simulink model "sampleModel283"  (R2021b)
settings: Solver=VariableStepAuto  StartTime=0.0  StopTime=10.0  RelTol=1e-3
undefined symbols (not defined in the file or in its folder): DiscIntNeverNeededParam
libraries: simulink x9, slpidlib x3
settings Model: Creator=user  LastModifiedBy=user

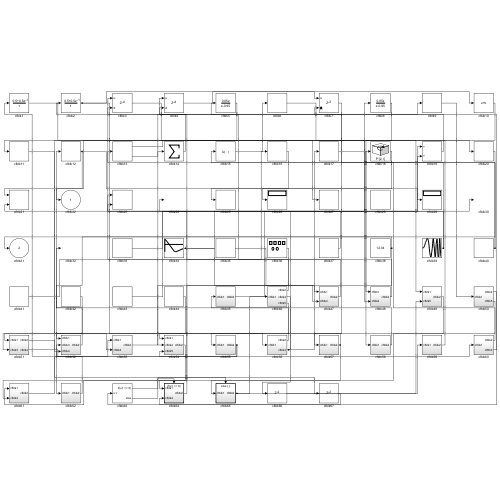
[thumbnail: Simulink's stored preview of the top-level diagram]
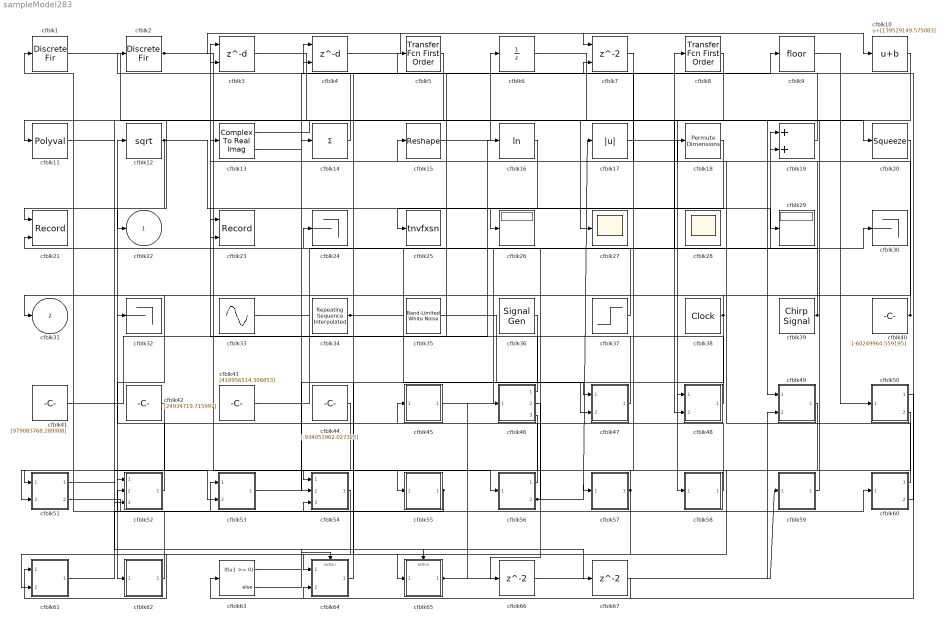
== system sampleModel283 ==
  cfblk1 : DiscreteFir  SampleTime=1
  cfblk10 : Bias  Bias=[139529149.575083]
  cfblk11 : Polyval  Coefs=[ +2.081618890e-019, -1.441693666e-014, +4.719686976e-010, -8.536869453e-006, +1.621573104e-001, -8.087801117e+001 ]
  cfblk12 : Sqrt  SaturateOnIntegerOverflow=on
  cfblk13 : ComplexToRealImag
  cfblk14 : Sum  Inputs=+
  cfblk15 : Reshape
  cfblk16 : Math  Operator=log  SaturateOnIntegerOverflow=on
  cfblk17 : Abs
  cfblk18 : PermuteDimensions
  cfblk19 : Sum
  cfblk2 : DiscreteFir  SampleTime=1
  cfblk20 : Squeeze
  cfblk21 : Record  FileSettingsInternal="{\"entries\":[{\"content\":{\"excelSettings\":{\"content\":{},\"type\":\"Streamout.ExcelSettings\"}},\"type\":\"Streamout.FileSettingStorage\",\"uuid\":\"8694a5bb-1d16-4ad7-950e-c35a4b4d7b5d\"}],\"packageUris\":[\"http://schema.mathworks.com/mf0/streamout_blocks/R2020a\"],\"version\":\"1.0\"}"  Layout=[1 1]  SignalsInternal="{\"entries\":[{\"content\":{\"signals\":[{\"content\":{\"blockPath\":[\"sampleModel283/cfblk21\"],\"channel\":[],\"dimensions\":[1],\"domain\":\"sampleModel283/cfblk21\",\"lineColor\":\"#a2142f\",\"plots\":[1],\"port\":1,\"sid\":[\"\"],\"signalID\":12100,\"signalName\":\"cfblk12\"},\"type\":\"RecordBlkView.Signal\",\"uuid\":\"68d03bc7-fcef-4d0a-a321-f31d8b845c33\"},{\"content\":{\"blockPath\":[\"sampleModel283/cfblk21\"],\"channel\":[],\"dimensions\":[1],\"domain\":\"sampleModel283/cfblk21\",\"lineColor\":\"#139fff\",\"plots\":[1],\"port\":2,\"sid\":[\"\"],\"signalID\":12104,\"signalName\":\"cfblk37\"},\"type\":\"RecordBlkView.Signal\",\"uuid\":\"b222a0ad-5142-49e8-822e-f4ea90e28b72\"}]},\"type\":\"RecordBlkView.InputSignals\",\"uuid\":\"76179848-0323-487f-86f4-e1829027746c\"}],\"packageUris\":[\"http://schema.mathworks.com/mf0/streamout_blocks/R2020a\"],\"version\":\"1.0\"}"  VisualizationBindings="{\"xyplotplugin\":{\"info\":[{\"series\":[{\"bindingParametersList\":[{\"parameter\":\"X-Axis\",\"signalID\":12100,\"signalName\":\"cfblk12\"},{\"parameter\":\"Y-Axis\",\"signalID\":12104,\"signalName\":\"cfblk37\"}],\"seriesID\":11155}],\"subplotID\":1}]}}"  CompatibilityTag=XY
  cfblk23 : Record  FileSettingsInternal="{\"entries\":[{\"content\":{\"excelSettings\":{\"content\":{},\"type\":\"Streamout.ExcelSettings\"}},\"type\":\"Streamout.FileSettingStorage\",\"uuid\":\"90ddd849-edd4-4e39-a333-4208290193cd\"}],\"packageUris\":[\"http://schema.mathworks.com/mf0/streamout_blocks/R2020a\"],\"version\":\"1.0\"}"  Layout=[1 1]  SignalsInternal="{\"entries\":[{\"content\":{\"signals\":[{\"content\":{\"blockPath\":[\"sampleModel283/cfblk23\"],\"channel\":[],\"dimensions\":[1],\"domain\":\"sampleModel283/cfblk23\",\"lineColor\":\"#a2142f\",\"plots\":[1],\"port\":1,\"sid\":[\"\"],\"signalID\":12108,\"signalName\":\"cfblk39\"},\"type\":\"RecordBlkView.Signal\",\"uuid\":\"9c057a92-301d-4b39-ab38-061aa18ef5d9\"},{\"content\":{\"blockPath\":[\"sampleModel283/cfblk23\"],\"channel\":[],\"dimensions\":[1],\"domain\":\"sampleModel283/cfblk23\",\"lineColor\":\"#139fff\",\"plots\":[1],\"port\":2,\"sid\":[\"\"],\"signalID\":12112,\"signalName\":\"cfblk56:2\"},\"type\":\"RecordBlkView.Signal\",\"uuid\":\"a825d14d-2c29-4b3e-948f-2c2b4e7bd86f\"}]},\"type\":\"RecordBlkView.InputSignals\",\"uuid\":\"38af6987-c0c5-4704-b1ef-83ad3136d3ff\"}],\"packageUris\":[\"http://schema.mathworks.com/mf0/streamout_blocks/R2020a\"],\"version\":\"1.0\"}"  VisualizationBindings="{\"xyplotplugin\":{\"info\":[{\"series\":[{\"bindingParametersList\":[{\"parameter\":\"X-Axis\",\"signalID\":12108,\"signalName\":\"cfblk39\"},{\"parameter\":\"Y-Axis\",\"signalID\":12112,\"signalName\":\"cfblk56:2\"}],\"seriesID\":64880}],\"subplotID\":1}]}}"  CompatibilityTag=XY
  cfblk24 : Terminator
  cfblk25 : ToWorkspace  VariableName=tnvfxsn  SaveFormat=Timeseries  SampleTime=-1
  cfblk26 : Display
  cfblk27 : Scope
  cfblk28 : Scope
      settings: Floating=on
  cfblk29 : Display
  cfblk3 : Delay  DelayLengthSource=Input port  SampleTime=1
      settings: InputPortMap=u0,p1
  cfblk30 : Terminator
  cfblk32 : Terminator
  cfblk33 : Sin  Amplitude=[128819876.540734]  Bias=[698200433.289732]  SampleTime=0
  cfblk34 : simulink/Sources/Repeating Sequence Interpolated  OutValues=[457661850.297885, 290690144.508280, -581221308.548181, -642320160.638465, -356637687.568462]  TimeValues=[0 0.1 0.5 0.6 1].'  LookUpMeth=Use Input Below  tsamp=0.01  OutMin=[]  OutMax=[]  OutDataTypeStr=double  OutputDataTypeScalingMode=double  OutDataType=fixdt(0,8)  OutScaling=2^-10
  cfblk35 : simulink/Sources/Band-Limited White Noise  Cov=[1006841987.893803]  Ts=0.1  seed=[5581259503.000000]
  cfblk36 : SignalGenerator  WaveForm=square  Amplitude=[368174655.835128]  Units=rad/sec
  cfblk37 : Step  Time=[38.000000]  Before=[-937039488.309373]  After=[-569842712.243944]  SampleTime=0
  cfblk38 : DigitalClock
  cfblk39 : simulink/Sources/Chirp Signal  f1=[685027736.106860]  T=[-403921099.241479]  f2=[736095362.275255]
  cfblk4 : Delay  DelayLengthSource=Input port  SampleTime=1
      settings: InputPortMap=u0,p1
  cfblk40 : Constant  Value=[-60249964.559195]  SampleTime=1
  cfblk41 : Constant  Value=[979083768.289908]  SampleTime=1
  cfblk42 : Constant  Value=[24934719.715997]  SampleTime=1
  cfblk43 : Constant  Value=[418956514.306853]  SampleTime=1
  cfblk44 : Constant  Value=[-934051962.027325]  SampleTime=1
  cfblk45 : Subsystem
  cfblk46 : Subsystem
  cfblk47 : Subsystem
  cfblk48 : Subsystem
  cfblk49 : Subsystem
  cfblk5 : simulink/Discrete/Transfer Fcn First Order  PoleZ=0.95  ICPrevOutput=0.0  DoSatur=off
  cfblk50 : Subsystem
  cfblk51 : Subsystem
  cfblk52 : Subsystem
  cfblk53 : Subsystem
  cfblk54 : Subsystem
  cfblk55 : Subsystem
  cfblk56 : Subsystem
  cfblk57 : Subsystem
  cfblk58 : Subsystem
  cfblk59 : Subsystem
  cfblk6 : UnitDelay  HasFrameUpgradeWarning=on
  cfblk60 : Subsystem
  cfblk61 : Subsystem
  cfblk62 : Subsystem
  cfblk63 : If  IfExpression=u1 >= 0  SampleTime=1
  cfblk64 : Subsystem  TreatAsAtomicUnit=on
  cfblk65 : Subsystem  TreatAsAtomicUnit=on
  cfblk66 : Delay  SampleTime=1
  cfblk67 : Delay  SampleTime=1
  cfblk7 : Delay  ShowEnablePort=on  SampleTime=1
      settings: InputPortMap=u0,e6
  cfblk8 : simulink/Discrete/Transfer Fcn First Order  PoleZ=0.95  ICPrevOutput=0.0  DoSatur=off
  cfblk9 : Rounding
  cfblk22 : Outport
  cfblk31 : Outport  Port=2
  wires:
  cfblk18/1 -> cfblk25/1
  cfblk17/1 -> cfblk58/1(cfblk1)
  cfblk44/1 -> cfblk54/1(cfblk1)
  cfblk49/1(cfblk2) -> cfblk65/1(cfblk1)
  cfblk12/1 -> cfblk21/1, cfblk29/1
  cfblk59/1(cfblk2) -> cfblk11/1
  cfblk2/1 -> cfblk56/1(cfblk1), cfblk7/1
  cfblk9/1 -> cfblk50/1(cfblk1)
  cfblk45/1(cfblk2) -> cfblk30/1
  cfblk50/1(cfblk2) -> cfblk63/1
  cfblk4/1 -> cfblk10/1
  cfblk56/1(cfblk2) -> cfblk45/1(cfblk1)
  cfblk53/1(cfblk2) -> cfblk14/1
  cfblk42/1 -> cfblk62/1(cfblk1)
  cfblk52/1(cfblk2) -> cfblk12/1
  cfblk58/1(cfblk2) -> cfblk32/1
  cfblk47/1(cfblk2) -> cfblk3/1
  cfblk56/2(cfblk4) -> cfblk17/1, cfblk23/2
  cfblk54/1(cfblk2) -> cfblk61/1(cfblk1)
  cfblk46/1(cfblk2) -> cfblk4/1
  cfblk33/1 -> cfblk19/1
  cfblk8/1 -> cfblk48/1(cfblk1)
  cfblk7/1 -> cfblk57/1(cfblk1)
  cfblk34/1 -> cfblk19/2, cfblk47/2(cfblk4)
  cfblk36/1 -> cfblk64/1(cfblk1)
  cfblk60/1(cfblk2) -> cfblk18/1
  cfblk40/1 -> cfblk13/1, cfblk7/2
  cfblk64/1(cfblk2) -> cfblk24/1
  cfblk15/1 -> cfblk6/1
  cfblk16/1 -> cfblk26/1
  cfblk65/1(cfblk2) -> cfblk59/1(cfblk1), cfblk46/1(cfblk1)
  cfblk61/1(cfblk2) -> cfblk60/1(cfblk1)
  cfblk6/1 -> cfblk49/1(cfblk1)
  cfblk57/1(cfblk2) -> cfblk51/1(cfblk1), cfblk61/2(cfblk4)
  cfblk37/1 -> cfblk21/2
  cfblk1/1 -> cfblk48/2(cfblk4)
  cfblk38/1 -> cfblk31/1, cfblk54/2(cfblk4)
  cfblk20/1 -> cfblk52/1(cfblk1)
  cfblk3/1 -> cfblk27/1
  cfblk51/2(cfblk4) -> cfblk53/1(cfblk1)
  cfblk5/1 -> cfblk22/1
  cfblk55/1(cfblk2) -> cfblk52/2(cfblk3), cfblk54/3(cfblk5)
  cfblk48/1(cfblk2) -> cfblk15/1
  cfblk11/1 -> cfblk53/2(cfblk4)
  cfblk14/1 -> cfblk4/2
  cfblk60/2(cfblk3) -> cfblk3/2
  cfblk62/1(cfblk2) -> cfblk1/1
  cfblk19/1 -> cfblk2/1
  cfblk43/1 -> cfblk8/1
  cfblk46/3(cfblk5) -> cfblk51/2(cfblk3)
  cfblk41/1 -> cfblk16/1
  cfblk50/2(cfblk5) -> cfblk55/1(cfblk1)
  cfblk10/1 -> cfblk52/3(cfblk4)
  cfblk13/1 -> cfblk20/1
  cfblk39/1 -> cfblk23/1, cfblk5/1
  cfblk35/1 -> cfblk47/1(cfblk1)
  cfblk13/2 -> cfblk9/1
  cfblk63/1 -> cfblk64/Action
  cfblk63/2 -> cfblk65/Action
  cfblk46/2(cfblk4) -> cfblk66/1
  cfblk66/1 -> cfblk49/2(cfblk5)
  cfblk51/1(cfblk2) -> cfblk67/1
  cfblk67/1 -> cfblk64/2(cfblk4)

== system sampleModel283/cfblk45 ==
  cfblk1 : Inport
  cfblk3 : DiscreteFir  SampleTime=1
  cfblk2 : Outport
  wires:
  cfblk1/1 -> cfblk3/1
  cfblk3/1 -> cfblk2/1

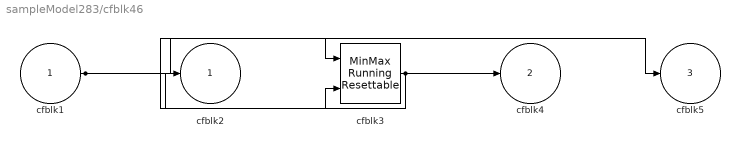
== system sampleModel283/cfblk46 ==
  cfblk1 : Inport
  cfblk3 : simulink/Math Operations/MinMax Running Resettable  Function=min  vinit=0.0
  cfblk2 : Outport
  cfblk4 : Outport  Port=2
  cfblk5 : Outport  Port=3
  wires:
  cfblk1/1 -> cfblk3/1, cfblk3/2, cfblk5/1
  cfblk3/1 -> cfblk2/1, cfblk4/1

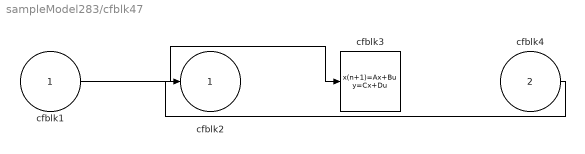
== system sampleModel283/cfblk47 ==
  cfblk1 : Inport
  cfblk4 : Inport  Port=2
  cfblk3 : DiscreteStateSpace
  cfblk2 : Outport
  wires:
  cfblk1/1 -> cfblk3/1
  cfblk4/1 -> cfblk2/1

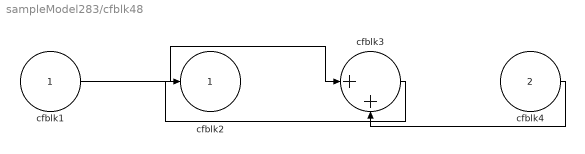
== system sampleModel283/cfblk48 ==
  cfblk1 : Inport
  cfblk4 : Inport  Port=2
  cfblk3 : Sum  Inputs=|++
  cfblk2 : Outport
  wires:
  cfblk1/1 -> cfblk3/1
  cfblk3/1 -> cfblk2/1
  cfblk4/1 -> cfblk3/2

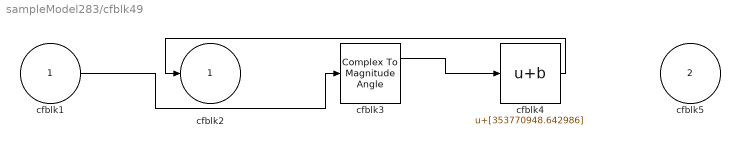
== system sampleModel283/cfblk49 ==
  cfblk1 : Inport
  cfblk5 : Inport  Port=2
  cfblk3 : ComplexToMagnitudeAngle
  cfblk4 : Bias  Bias=[353770948.642986]
  cfblk2 : Outport
  wires:
  cfblk4/1 -> cfblk2/1
  cfblk1/1 -> cfblk3/1
  cfblk3/1 -> cfblk4/1

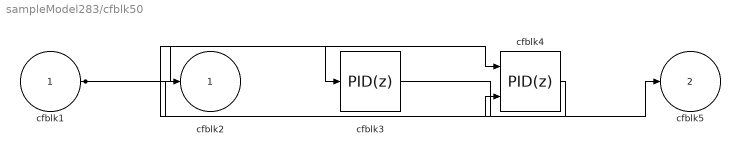
== system sampleModel283/cfblk50 ==
  cfblk1 : Inport
  cfblk3 : slpidlib/PID Controller  Controller=PID  Form=Parallel  TimeDomain=Discrete-time  UseExternalTs=off  SampleTime=1  IntegratorMethod=Forward Euler  FilterMethod=Forward Euler  ControllerParametersSource=internal  P=1  I=1  D=0  UseFilter=on  N=100  TunerSelectOption=Transfer Function Based (PID Tuner App)  InitialConditionSource=internal  InitialConditionForIntegrator=0  InitialConditionForFilter=0  DifferentiatorICPrevScaledInput=0  ExternalReset=none  TrackingMode=off  Kt=1  LimitOutput=off  SatLimitsSource=internal  UpperSaturationLimit=inf  LowerSaturationLimit=-inf  LinearizeAsGain=off  AntiWindupMode=none  Kb=1  POutMin=[]  POutMax=[]  IOutMin=[]  IOutMax=[]  DOutMin=[]  DOutMax=[]  NOutMin=[]  NOutMax=[]  SumOutMin=[]  SumOutMax=[]  SaturationOutMin=[]  SaturationOutMax=[]  PParamMin=[]  PParamMax=[]  IParamMin=[]  IParamMax=[]  DParamMin=[]  DParamMax=[]  NParamMin=[]  NParamMax=[]  KbParamMin=[]  KbParamMax=[]  KtParamMin=[]  KtParamMax=[]  KbOutMin=[]  KbOutMax=[]  KtOutMin=[]  KtOutMax=[]  IntegratorOutMin=[]  IntegratorOutMax=[]  FilterOutMin=[]  FilterOutMax=[]  SumI1OutMin=[]  SumI1OutMax=[]  SumI2OutMin=[]  SumI2OutMax=[]  SumI3OutMin=[]  SumI3OutMax=[]  SumI4OutMin=[]  SumI4OutMax=[]  SumDOutMin=[]  SumDOutMax=[]  DifferentiatorOutMin=[]  DifferentiatorOutMax=[]  FilterDiffOutCoefMin=[]  FilterDiffOutCoefMax=[]  ReciprocalOutMin=[]  ReciprocalOutMax=[]  SumDenOutMin=[]  SumDenOutMax=[]  SumNumOutMin=[]  SumNumOutMax=[]  DivideOutMin=[]  DivideOutMax=[]  UdiffTsProdOutMin=[]  UdiffTsProdOutMax=[]  NTsProdOutMin=[]  NTsProdOutMax=[]  UintegralTsProdOutMin=[]  UintegralTsProdOutMax=[]  UngainTsProdOutMin=[]  UngainTsProdOutMax=[]  IntegratorContinuousStateAttributes=''  IntegratorStateMustResolveToSignalObject=off  IntegratorRTWStateStorageClass=Auto  FilterContinuousStateAttributes=''  FilterStateMustResolveToSignalObject=off  FilterRTWStateStorageClass=Auto  ParallelPVariant=InternalParameters  IdealPVariant=Disabled  IVariant=InternalParameters  DVariant=InternalParameters  IntegratorVariant=Discrete  SatVariant=Disabled  AWVariant=Passthrough  PCopyVariant=Disabled  TRVariant=Disabled  FdbkBlocksVariant=Forward  IdealPFdbkVariant=Disabled  SatFdbkVariant=Disabled  DerivativeFilterVariant=ForwardEulerFilter  NVariant=InternalParameters  NCopyVariant=Disabled  FilterICVariant=InternalICsFilter  IntegratorICVariant=InternalICs  ExternalResetVariant=Disabled  TRSumVariant=Passthrough  SumFdbkVariant=Disabled  SumVariant=Sum_PID  TsampFilterVariant=InternalTs  TsampNgainVariant=Passthrough  TsampIntegralVariant=Passthrough  ExternalSaturationOutDataTypeStr=Inherit: Same as second input
  cfblk4 : slpidlib/PID Controller (2DOF)  Controller=PID  Form=Parallel  TimeDomain=Discrete-time  UseExternalTs=off  SampleTime=1  IntegratorMethod=Forward Euler  FilterMethod=Forward Euler  ControllerParametersSource=internal  P=1  I=1  D=0  UseFilter=on  N=100  b=1  c=1  TunerSelectOption=Transfer Function Based (PID Tuner App)  InitialConditionSource=internal  InitialConditionForIntegrator=0  InitialConditionForFilter=0  DifferentiatorICPrevScaledInput=0  ExternalReset=none  TrackingMode=off  Kt=1  LimitOutput=off  SatLimitsSource=internal  UpperSaturationLimit=inf  LowerSaturationLimit=-inf  LinearizeAsGain=off  AntiWindupMode=none  Kb=1  POutMin=[]  POutMax=[]  IOutMin=[]  IOutMax=[]  DOutMin=[]  DOutMax=[]  NOutMin=[]  NOutMax=[]  bOutMin=[]  bOutMax=[]  cOutMin=[]  cOutMax=[]  SumOutMin=[]  SumOutMax=[]  SaturationOutMin=[]  SaturationOutMax=[]  PParamMin=[]  PParamMax=[]  IParamMin=[]  IParamMax=[]  DParamMin=[]  DParamMax=[]  NParamMin=[]  NParamMax=[]  bParamMin=[]  bParamMax=[]  cParamMin=[]  cParamMax=[]  KbParamMin=[]  KbParamMax=[]  KtParamMin=[]  KtParamMax=[]  KbOutMin=[]  KbOutMax=[]  KtOutMin=[]  KtOutMax=[]  IntegratorOutMin=[]  IntegratorOutMax=[]  FilterOutMin=[]  FilterOutMax=[]  SumI1OutMin=[]  SumI1OutMax=[]  SumI2OutMin=[]  SumI2OutMax=[]  SumI3OutMin=[]  SumI3OutMax=[]  SumI4OutMin=[]  SumI4OutMax=[]  SumDOutMin=[]  SumDOutMax=[]  Sum1OutMin=[]  Sum1OutMax=[]  Sum2OutMin=[]  Sum2OutMax=[]  Sum3OutMin=[]  Sum3OutMax=[]  DifferentiatorOutMin=[]  DifferentiatorOutMax=[]  FilterDiffOutCoefMin=[]  FilterDiffOutCoefMax=[]  ReciprocalOutMin=[]  ReciprocalOutMax=[]  SumDenOutMin=[]  SumDenOutMax=[]  SumNumOutMin=[]  SumNumOutMax=[]  DivideOutMin=[]  DivideOutMax=[]  UdiffTsProdOutMin=[]  UdiffTsProdOutMax=[]  NTsProdOutMin=[]  NTsProdOutMax=[]  UintegralTsProdOutMin=[]  UintegralTsProdOutMax=[]  UngainTsProdOutMin=[]  UngainTsProdOutMax=[]  IntegratorContinuousStateAttributes=''  IntegratorStateMustResolveToSignalObject=off  IntegratorRTWStateStorageClass=Auto  FilterContinuousStateAttributes=''  FilterStateMustResolveToSignalObject=off  FilterRTWStateStorageClass=Auto  ParallelPVariant=InternalParameters  IdealPVariant=Disabled  IVariant=InternalParameters  DVariant=InternalParameters  bVariant=InternalParameters  cVariant=InternalParameters  IntegratorVariant=Discrete  SatVariant=Disabled  AWVariant=Passthrough  PCopyVariant=Disabled  TRVariant=Disabled  FdbkBlocksVariant=Forward  IdealPFdbkVariant=Disabled  SatFdbkVariant=Disabled  DerivativeFilterVariant=ForwardEulerFilter  NVariant=InternalParameters  NCopyVariant=Disabled  FilterICVariant=InternalICsFilter  IntegratorICVariant=InternalICs  ExternalResetVariant=Disabled  TRSumVariant=Passthrough  SumFdbkVariant=Disabled  SumVariant=Sum_PID  TsampFilterVariant=InternalTs  TsampNgainVariant=Passthrough  TsampIntegralVariant=Passthrough  ExternalSaturationOutDataTypeStr=Inherit: Same as second input
      settings: SourceProductBaseCode=SL
  cfblk2 : Outport
  cfblk5 : Outport  Port=2
  wires:
  cfblk1/1 -> cfblk4/1, cfblk3/1, cfblk4/2
  cfblk4/1 -> cfblk2/1
  cfblk3/1 -> cfblk5/1

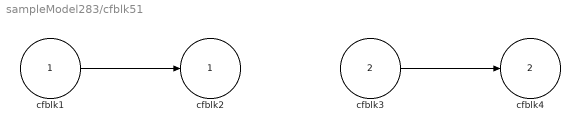
== system sampleModel283/cfblk51 ==
  cfblk1 : Inport
  cfblk3 : Inport  Port=2
  cfblk2 : Outport
  cfblk4 : Outport  Port=2
  wires:
  cfblk3/1 -> cfblk4/1
  cfblk1/1 -> cfblk2/1

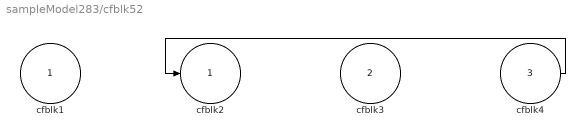
== system sampleModel283/cfblk52 ==
  cfblk1 : Inport
  cfblk3 : Inport  Port=2
  cfblk4 : Inport  Port=3
  cfblk2 : Outport
  wires:
  cfblk4/1 -> cfblk2/1

== system sampleModel283/cfblk53 ==
  cfblk1 : Inport
  cfblk4 : Inport  Port=2
  cfblk3 : Product  Inputs=*
  cfblk2 : Outport
  wires:
  cfblk4/1 -> cfblk3/1
  cfblk3/1 -> cfblk2/1

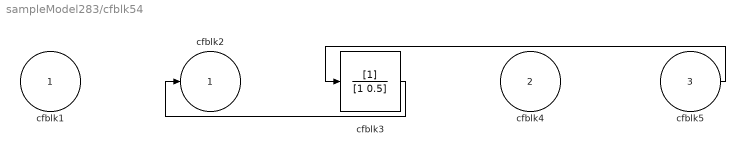
== system sampleModel283/cfblk54 ==
  cfblk1 : Inport
  cfblk4 : Inport  Port=2
  cfblk5 : Inport  Port=3
  cfblk3 : DiscreteFilter  SampleTime=1
  cfblk2 : Outport
  wires:
  cfblk5/1 -> cfblk3/1
  cfblk3/1 -> cfblk2/1

== system sampleModel283/cfblk55 ==
  cfblk1 : Inport
  cfblk3 : simulink/Discrete/Transfer Fcn Lead or Lag  PoleZ=0.95  ZeroZ=0.75  ICPrevOutput=0.0  ICPrevInput=0.0  DoSatur=off
      settings: SourceProductBaseCode=SL
  cfblk4 : ComplexToRealImag
  cfblk2 : Outport
  wires:
  cfblk1/1 -> cfblk3/1
  cfblk4/1 -> cfblk2/1
  cfblk3/1 -> cfblk4/1

== system sampleModel283/cfblk56 ==
  cfblk1 : Inport
  cfblk3 : Constant  Value=[388963075.985211]  SampleTime=1
  cfblk2 : Outport
  cfblk4 : Outport  Port=2
  wires:
  cfblk3/1 -> cfblk2/1
  cfblk1/1 -> cfblk4/1

== system sampleModel283/cfblk57 ==
  cfblk1 : Inport
  cfblk3 : slpidlib/PID Controller (2DOF)  Controller=PID  Form=Parallel  TimeDomain=Discrete-time  UseExternalTs=off  SampleTime=1  IntegratorMethod=Forward Euler  FilterMethod=Forward Euler  ControllerParametersSource=internal  P=1  I=1  D=0  UseFilter=on  N=100  b=1  c=1  TunerSelectOption=Transfer Function Based (PID Tuner App)  InitialConditionSource=internal  InitialConditionForIntegrator=0  InitialConditionForFilter=0  DifferentiatorICPrevScaledInput=0  ExternalReset=none  TrackingMode=off  Kt=1  LimitOutput=off  SatLimitsSource=internal  UpperSaturationLimit=inf  LowerSaturationLimit=-inf  LinearizeAsGain=off  AntiWindupMode=none  Kb=1  POutMin=[]  POutMax=[]  IOutMin=[]  IOutMax=[]  DOutMin=[]  DOutMax=[]  NOutMin=[]  NOutMax=[]  bOutMin=[]  bOutMax=[]  cOutMin=[]  cOutMax=[]  SumOutMin=[]  SumOutMax=[]  SaturationOutMin=[]  SaturationOutMax=[]  PParamMin=[]  PParamMax=[]  IParamMin=[]  IParamMax=[]  DParamMin=[]  DParamMax=[]  NParamMin=[]  NParamMax=[]  bParamMin=[]  bParamMax=[]  cParamMin=[]  cParamMax=[]  KbParamMin=[]  KbParamMax=[]  KtParamMin=[]  KtParamMax=[]  KbOutMin=[]  KbOutMax=[]  KtOutMin=[]  KtOutMax=[]  IntegratorOutMin=[]  IntegratorOutMax=[]  FilterOutMin=[]  FilterOutMax=[]  SumI1OutMin=[]  SumI1OutMax=[]  SumI2OutMin=[]  SumI2OutMax=[]  SumI3OutMin=[]  SumI3OutMax=[]  SumI4OutMin=[]  SumI4OutMax=[]  SumDOutMin=[]  SumDOutMax=[]  Sum1OutMin=[]  Sum1OutMax=[]  Sum2OutMin=[]  Sum2OutMax=[]  Sum3OutMin=[]  Sum3OutMax=[]  DifferentiatorOutMin=[]  DifferentiatorOutMax=[]  FilterDiffOutCoefMin=[]  FilterDiffOutCoefMax=[]  ReciprocalOutMin=[]  ReciprocalOutMax=[]  SumDenOutMin=[]  SumDenOutMax=[]  SumNumOutMin=[]  SumNumOutMax=[]  DivideOutMin=[]  DivideOutMax=[]  UdiffTsProdOutMin=[]  UdiffTsProdOutMax=[]  NTsProdOutMin=[]  NTsProdOutMax=[]  UintegralTsProdOutMin=[]  UintegralTsProdOutMax=[]  UngainTsProdOutMin=[]  UngainTsProdOutMax=[]  IntegratorContinuousStateAttributes=''  IntegratorStateMustResolveToSignalObject=off  IntegratorRTWStateStorageClass=Auto  FilterContinuousStateAttributes=''  FilterStateMustResolveToSignalObject=off  FilterRTWStateStorageClass=Auto  ParallelPVariant=InternalParameters  IdealPVariant=Disabled  IVariant=InternalParameters  DVariant=InternalParameters  bVariant=InternalParameters  cVariant=InternalParameters  IntegratorVariant=Discrete  SatVariant=Disabled  AWVariant=Passthrough  PCopyVariant=Disabled  TRVariant=Disabled  FdbkBlocksVariant=Forward  IdealPFdbkVariant=Disabled  SatFdbkVariant=Disabled  DerivativeFilterVariant=ForwardEulerFilter  NVariant=InternalParameters  NCopyVariant=Disabled  FilterICVariant=InternalICsFilter  IntegratorICVariant=InternalICs  ExternalResetVariant=Disabled  TRSumVariant=Passthrough  SumFdbkVariant=Disabled  SumVariant=Sum_PID  TsampFilterVariant=InternalTs  TsampNgainVariant=Passthrough  TsampIntegralVariant=Passthrough  ExternalSaturationOutDataTypeStr=Inherit: Same as second input
      settings: SourceProductBaseCode=SL
  cfblk4 : Sum  Inputs=--
  cfblk2 : Outport
  wires:
  cfblk3/1 -> cfblk4/1
  cfblk1/1 -> cfblk4/2, cfblk3/1, cfblk3/2
  cfblk4/1 -> cfblk2/1

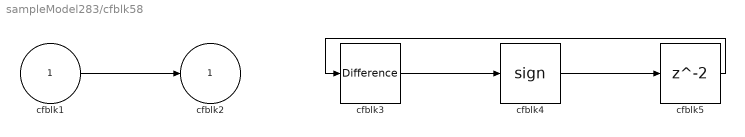
== system sampleModel283/cfblk58 ==
  cfblk1 : Inport
  cfblk3 : simulink/Discrete/Difference  ICPrevInput=0.0  OutMin=[]  OutMax=[]  OutDataTypeStr=Inherit: Inherit via back propagation  OutDataType=fixdt(1, 16)  OutScaling=2^-10  DoSatur=off
  cfblk4 : Signum
  cfblk5 : Delay  SampleTime=1
  cfblk2 : Outport
  wires:
  cfblk3/1 -> cfblk4/1
  cfblk1/1 -> cfblk2/1
  cfblk4/1 -> cfblk5/1
  cfblk5/1 -> cfblk3/1

== system sampleModel283/cfblk59 ==
  cfblk1 : Inport
  cfblk3 : Math  Operator=transpose  SaturateOnIntegerOverflow=on
  cfblk2 : Outport
  wires:
  cfblk1/1 -> cfblk2/1, cfblk3/1

== system sampleModel283/cfblk60 ==
  cfblk1 : Inport
  cfblk2 : Outport
  cfblk3 : Outport  Port=2
  wires:
  cfblk1/1 -> cfblk3/1, cfblk2/1

== system sampleModel283/cfblk61 ==
  cfblk1 : Inport
  cfblk4 : Inport  Port=2
  cfblk3 : DiscreteIntegrator  ICPrevOutput=DiscIntNeverNeededParam  ICPrevScaledInput=DiscIntNeverNeededParam
  cfblk2 : Outport
  wires:
  cfblk1/1 -> cfblk3/1
  cfblk3/1 -> cfblk2/1

== system sampleModel283/cfblk62 ==
  cfblk1 : Inport
  cfblk3 : Trigonometry
  cfblk2 : Outport
  wires:
  cfblk1/1 -> cfblk3/1
  cfblk3/1 -> cfblk2/1

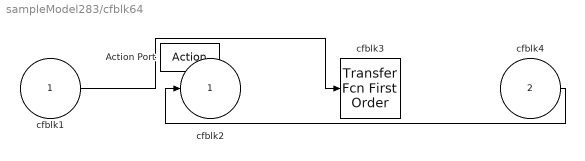
== system sampleModel283/cfblk64 ==
  cfblk1 : Inport
  cfblk4 : Inport  Port=2
  Action Port : ActionPort  ActionPortLabel=if(u1 >= 0)
  cfblk3 : simulink/Discrete/Transfer Fcn First Order  PoleZ=0.95  ICPrevOutput=0.0  DoSatur=off
  cfblk2 : Outport
  wires:
  cfblk4/1 -> cfblk2/1
  cfblk1/1 -> cfblk3/1

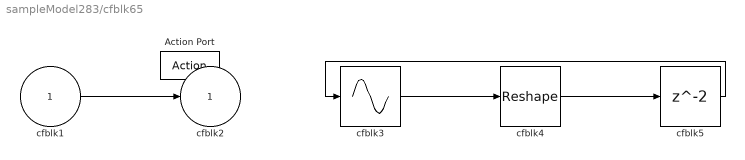
== system sampleModel283/cfblk65 ==
  cfblk1 : Inport
  Action Port : ActionPort  ActionPortLabel=else
  cfblk3 : Sin  TimeSource=Use external signal  SampleTime=0
  cfblk4 : Reshape
  cfblk5 : Delay
  cfblk2 : Outport
  wires:
  cfblk3/1 -> cfblk4/1
  cfblk1/1 -> cfblk2/1
  cfblk4/1 -> cfblk5/1
  cfblk5/1 -> cfblk3/1
